simulink model "FA_18_MPC_Single_Actuator"  (R2018a)
settings: Solver=ode45  StartTime=0.0  StopTime=120  RelTol=1e-3
PreLoadFcn:
  | F18_Linear
libraries: simulink_extras x11, mpclib x1
settings Model: Creator=User  LastModifiedBy=User
settings CodeAppCC: StateflowObjectComments=on

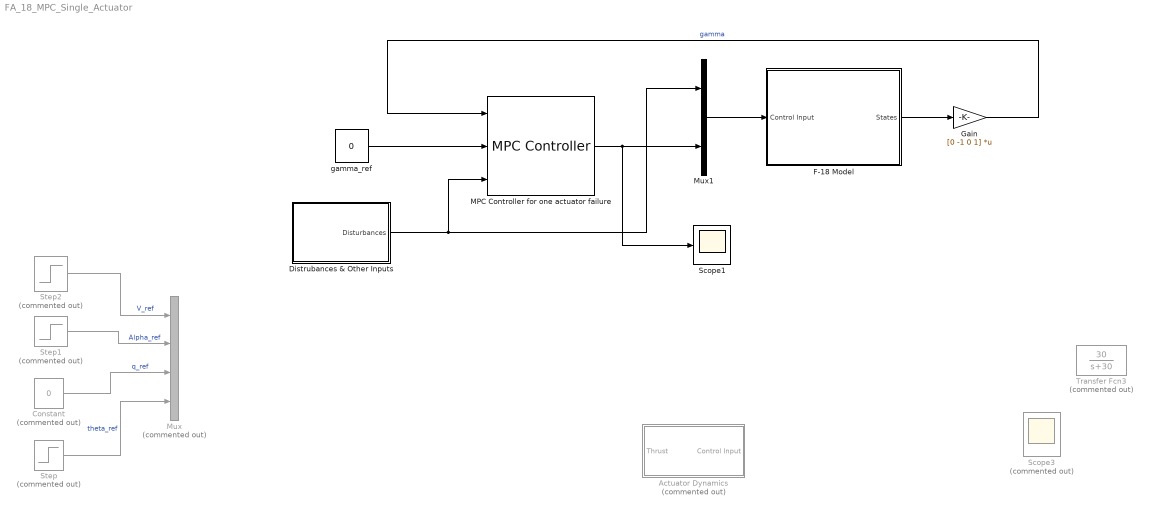
== system FA_18_MPC_Single_Actuator ==
  Actuator Dynamics : Subsystem  Commented=on
  Constant : Constant  Commented=on  Value=0
  Distrubances & Other Inputs : Subsystem
  F-18 Model : Subsystem
  Gain : Gain  Gain=[0 -1 0 1]  Multiplication=Matrix(K*u)
  MPC Controller for one actuator failure : mpclib/MPC Controller  SCDEnableBlockLinearizationSpecification=on  mpcobj=mpc1  is_multiple=0  enable_value=0  return_u0=off  updateMPCinCallerWorkspace=on  ref_from_ws=off  ref_signal_name=[]  ref_preview=off  md_from_ws=off  md_signal_name=[]  md_preview=off  from_project=off  project_file=MPCtask.mat  md_inport=on  mv_inport=off  cost_outport=off  return_sequence=off  return_qpstatus=off  return_state=off  state_inport=off  lims_inport=off  cc_inport=off  ywt_inport=off  is_designfromscratch=0  uwt_inport=off  duwt_inport=off  rhoeps_inport=off  uref_inport=off  n_ts=0.1  n_p=15  n_mv=1  n_md=3  n_ud=0  n_mo=1  n_uo=0  BlockDataType=double  SampleTimeInherited=off  switch_inport=off
  Mux : Mux  Commented=on
  Mux1 : Mux  Inputs=2
  Scope1 : Scope
  Scope3 : Scope  Commented=on
  Step : Step  Commented=on  SampleTime=0
  Step1 : Step  Commented=on  SampleTime=0
  Step2 : Step  Commented=on  After=50  SampleTime=0
  Transfer Fcn3 : TransferFcn  Commented=on  Numerator=[30]  Denominator=[1 30]
  gamma_ref : Constant  Value=0
  wires:
  F-18 Model/1(States) -> Gain/1
  Step1/1 -> Mux/2  "Alpha_ref"
  Step2/1 -> Mux/1  "V_ref"
  Constant/1 -> Mux/3  "q_ref"
  Step/1 -> Mux/4  "theta_ref"
  Gain/1 -> MPC Controller for one actuator failure/1  "gamma"
  Distrubances & Other Inputs/1(Disturbances) -> MPC Controller for one actuator failure/3, Mux1/1
  Mux1/1 -> F-18 Model/1(Control Input)
  gamma_ref/1 -> MPC Controller for one actuator failure/2
  MPC Controller for one actuator failure/1 -> Scope1/1, Mux1/2

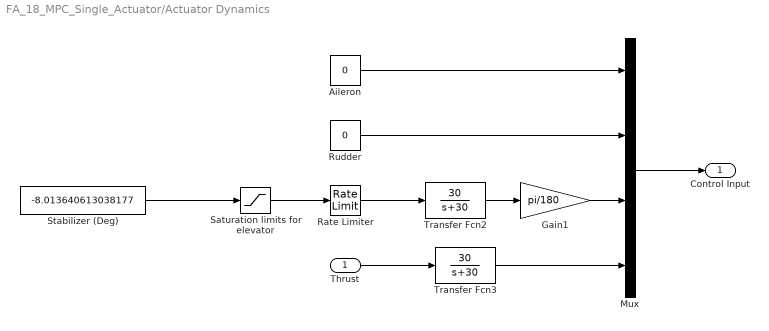
== system FA_18_MPC_Single_Actuator/Actuator Dynamics ==
  Thrust : Inport
  Aileron : Constant  Value=0
  Gain1 : Gain  Gain=pi/180
  Mux : Mux
  Rate Limiter : RateLimiter  RisingSlewLimit=40  FallingSlewLimit=-40  SampleTimeMode=inherited
  Rudder : Constant  Value=0
  Saturation limits for elevator : Saturate  UpperLimit=10.5  LowerLimit=-24
  Stabilizer (Deg) : Constant  Value=-8.013640613038177
  Transfer Fcn2 : TransferFcn  Numerator=[30]  Denominator=[1 30]
  Transfer Fcn3 : TransferFcn  Numerator=[30]  Denominator=[1 30]
  Control Input : Outport
  wires:
  Mux/1 -> Control Input/1
  Aileron/1 -> Mux/1
  Transfer Fcn3/1 -> Mux/4
  Rudder/1 -> Mux/2
  Thrust/1 -> Transfer Fcn3/1
  Saturation limits for elevator/1 -> Rate Limiter/1
  Rate Limiter/1 -> Transfer Fcn2/1
  Stabilizer (Deg)/1 -> Saturation limits for elevator/1
  Gain1/1 -> Mux/3
  Transfer Fcn2/1 -> Gain1/1

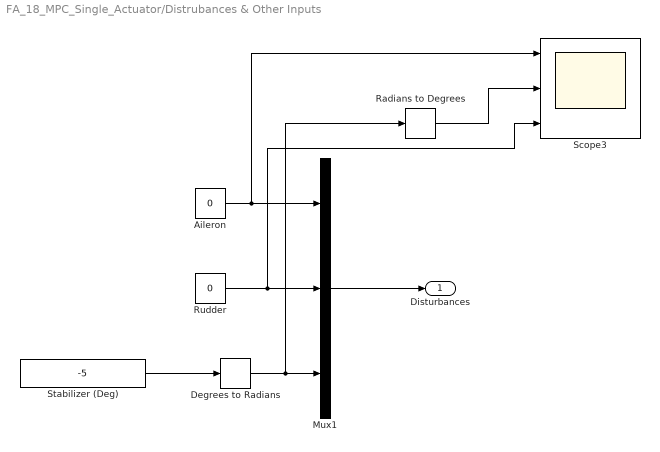
== system FA_18_MPC_Single_Actuator/Distrubances & Other Inputs ==
  Aileron : Constant  Value=0
  Degrees to Radians : simulink_extras/Transformations/Degrees to Radians
  Mux1 : Mux  Inputs=3
  Radians to Degrees : simulink_extras/Transformations/Radians to Degrees
  Rudder : Constant  Value=0
  Scope3 : Scope  NumInputPorts=3
  Stabilizer (Deg) : Constant  Value=-5
  Disturbances : Outport
  wires:
  Mux1/1 -> Disturbances/1
  Degrees to Radians/1 -> Radians to Degrees/1, Mux1/3
  Aileron/1 -> Scope3/1, Mux1/1
  Stabilizer (Deg)/1 -> Degrees to Radians/1
  Rudder/1 -> Scope3/3, Mux1/2
  Radians to Degrees/1 -> Scope3/2

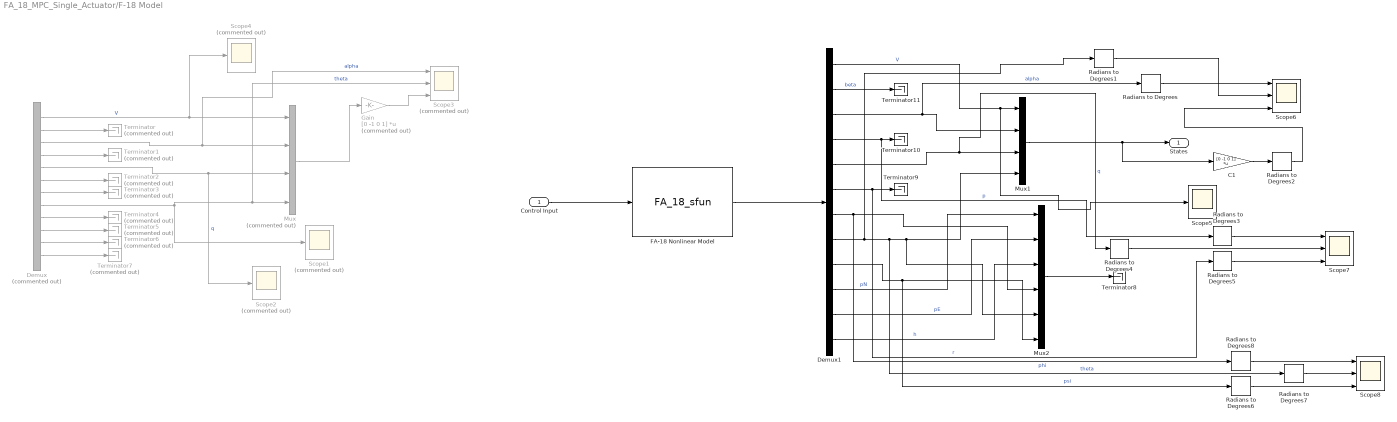
== system FA_18_MPC_Single_Actuator/F-18 Model ==
  Control Input : Inport
  C1 : Gain  Gain=[0 -1 0 1]  Multiplication=Matrix(K*u)
  Demux : Demux  Commented=on  Outputs=12
  Demux1 : Demux  Outputs=12
  FA-18 Nonlinear Model : S-Function  FunctionName=FA_18_sfun  SFunctionDeploymentMode=off  EnableBusSupport=off
  Gain : Gain  Commented=on  Gain=[0 -1 0 1]  Multiplication=Matrix(K*u)
  Mux : Mux  Commented=on
  Mux1 : Mux
  Mux2 : Mux  Inputs=6
  Radians to Degrees{,1..8} (9 alike) : simulink_extras/Transformations/Radians to Degrees
  Scope1 : Scope  Commented=on
  Scope2 : Scope  Commented=on
  Scope3 : Scope  Commented=on  NumInputPorts=3
  Scope4 : Scope  Commented=on
  Scope5 : Scope
  Scope6 : Scope  NumInputPorts=3
  Scope7 : Scope  NumInputPorts=3
  Scope8 : Scope  NumInputPorts=3
  Terminator{,1..7} (8 alike) : Terminator  Commented=on
  Terminator{8..11} (4 alike) : Terminator
  States : Outport
  wires:
  Control Input/1 -> FA-18 Nonlinear Model/1
  Demux/1 -> Scope4/1, Mux/1  "V"
  Demux/3 -> Scope3/1, Mux/2  "alpha"
  Demux/5 -> Scope2/1, Mux/3  "q"
  Demux/8 -> Scope1/1, Scope3/2, Mux/4  "theta"
  Demux/2 -> Terminator/1
  Demux/4 -> Terminator1/1
  Demux/6 -> Terminator2/1
  Demux/7 -> Terminator3/1
  Demux/9 -> Terminator4/1
  Demux/10 -> Terminator5/1
  Demux/11 -> Terminator6/1
  Demux/12 -> Terminator7/1
  Mux/1 -> Gain/1
  Gain/1 -> Scope3/3
  Radians to Degrees7/1 -> Scope8/2
  Demux1/4 -> Radians to Degrees3/1, Terminator10/1  "p"
  FA-18 Nonlinear Model/1 -> Demux1/1
  Radians to Degrees6/1 -> Scope8/3
  Demux1/11 -> Mux2/2  "pE"
  Demux1/5 -> Radians to Degrees4/1, Mux1/3  "q"
  Demux1/1 -> Scope5/1, Mux1/1  "V"
  Radians to Degrees8/1 -> Scope8/1
  Demux1/12 -> Mux2/3  "h"
  Demux1/10 -> Mux2/1  "pN"
  Demux1/2 -> Terminator11/1  "beta"
  Radians to Degrees3/1 -> Scope7/1
  Radians to Degrees2/1 -> Scope6/3
  Demux1/9 -> Radians to Degrees6/1, Mux2/6  "psi"
  Radians to Degrees1/1 -> Scope6/2
  Radians to Degrees4/1 -> Scope7/2
  Demux1/6 -> Radians to Degrees5/1, Terminator9/1  "r"
  Demux1/3 -> Radians to Degrees/1, Mux1/2  "alpha"
  Demux1/7 -> Radians to Degrees8/1, Mux2/4  "phi"
  Demux1/8 -> Radians to Degrees1/1, Radians to Degrees7/1, Mux2/5, Mux1/4  "theta"
  Mux2/1 -> Terminator8/1
  Radians to Degrees5/1 -> Scope7/3
  C1/1 -> Radians to Degrees2/1
  Mux1/1 -> C1/1, States/1
  Radians to Degrees/1 -> Scope6/1
